simulink model "ccc_core"  (Simulink 7.4)
settings: Solver=ode45  StartTime=0.0  StopTime=10000  RelTol=1e-3
libraries: xbsIndex_r4 x236, cfa_library x64, casper_library_misc x7
(part 2 of 5)

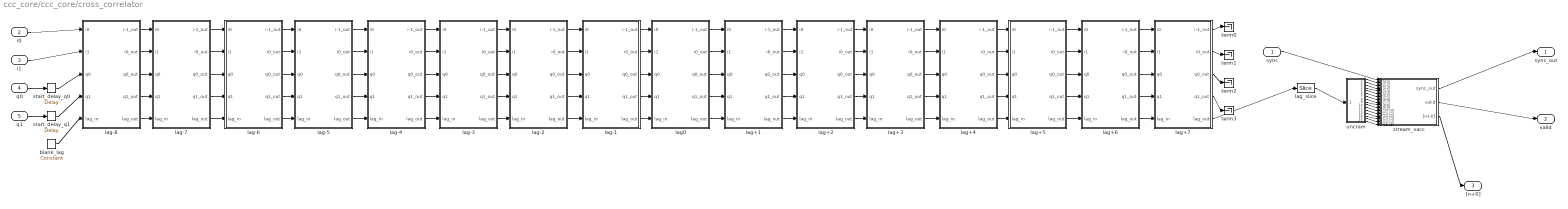
== system ccc_core/ccc_core/cross_correlator ==
  sync : Inport
  i0 : Inport  Port=2
  i1 : Inport  Port=3
  q0 : Inport  Port=4
  q1 : Inport  Port=5
  blank_lag : xbsIndex_r4/Constant  arith_type=Unsigned  const=0  n_bits=1  bin_pt=0  explicit_period=on  period=1  equ=P=C  opselect=C  inp2=PCIN>>17  opr=+  inp1=P  carry=CIN  dbl_ovrd=off  block_type=constant
  lag+1 : Subsystem  AncestorBlock=cfa_library/single_lag  mask(single_lag){n_inputs=1, specify_mult=off, mult_spec=Behavioral, specify_add=off, add_spec=Fabric, mult_delay=3, add_delay=2, overall_delay=2, use_2bit=on, complex_in=on, shift_q=off, shift_i=on}
      mask prompts: n_inputs "Number of Simultaneous Inputs: (2^?)"; specify_mult "Specify multiplier use (behavioural HDL if not specified)"; mult_spec "Multiplier specification:"; specify_add "Specify adder use (behavioural HDL if not specified)"; add_spec "Adder specification:"; mult_delay "Mult Latency:"; add_delay "Add Latency:"; overall_delay "Overall Latency:"; use_2bit "Use special 2-bit binary encoding"; complex_in "Complex inputs"; shift_q "Shift 'q' output"; shift_i "Shift 'i' output"
      mask help: This performs the computations for a single lag. Please use the 'cross_correlator' block to generate a full X-engine.
      mask init:
      | single_lag_init(gcb,...
      |     'n_inputs', n_inputs,...
      |     'specify_mult', specify_mult,...
      |     'mult_spec', mult_spec,...
      |     'specify_add', specify_add,...
      |     'add_spec', add_spec,...
      |     'mult_delay', mult_delay,...
      |     'add_delay', add_delay,...
      |     'overall_delay', overall_delay,...
      |     'use_2bit', use_2bit,...
      |     'complex_in', complex_in,...
      |     'shift_q', shift_q,...
      |     'shift_i', shift_i);
      settings: AttributesFormatString=|
      | Use 2-bit: on, Type: complex,
      |  Demux: 2, Add: Fabric,
      |  Mult: Behavioral
      mask StyleString: edit,checkbox,popup(Behavioral|Core|Embedded),checkbox,popup(Fabric|DSP48),edit,edit,edit,checkbox,checkbox,checkbox,checkbox
      mask CallbackString:
      | |specify_mult = get_param(gcb,'specify_mult');
      | enables = get_param(gcb, 'MaskEnables');
      | if( strcmp(specify_mult,'off')),
      |     enables{3} = 'off';
      | else,
      |     enables{3} = 'on';
      | end
      | set_param(gcb, 'MaskEnables', enables);
      | ||specify_add = get_param(gcb,'specify_add');
      | enables = get_param(gcb, 'MaskEnables');
      | if( strcmp(specify_add,'off')),
      |     enables{5} = 'off';
      | else,
      |     enables{5} = 'on';
      | end
      | set_param(gcb, 'MaskEnables', enables);
      | |||||use_2bit = get_param(gcb,'use_2bit');
      | enables = get_param(gcb, 'MaskEnables');
      | if( strcmp(use_2bit,'off')),
      |     enables{10} = 'off';
      | else,
      |     enables{10} = 'on';
      | end
      | set_param(gcb, 'MaskEnables', enables);|||
      mask TabNameString: Basic,Implementation,Implementation,Implementation,Implementation,Implementation,Implementation,Implementation,Basic,Basic,Basic,Basic
  lag+2 : Subsystem  AncestorBlock=cfa_library/single_lag  mask(single_lag){n_inputs=1, specify_mult=off, mult_spec=Behavioral, specify_add=off, add_spec=Fabric, mult_delay=3, add_delay=2, overall_delay=2, use_2bit=on, complex_in=on, shift_q=off, shift_i=on}
      mask prompts: n_inputs "Number of Simultaneous Inputs: (2^?)"; specify_mult "Specify multiplier use (behavioural HDL if not specified)"; mult_spec "Multiplier specification:"; specify_add "Specify adder use (behavioural HDL if not specified)"; add_spec "Adder specification:"; mult_delay "Mult Latency:"; add_delay "Add Latency:"; overall_delay "Overall Latency:"; use_2bit "Use special 2-bit binary encoding"; complex_in "Complex inputs"; shift_q "Shift 'q' output"; shift_i "Shift 'i' output"
      mask help: This performs the computations for a single lag. Please use the 'cross_correlator' block to generate a full X-engine.
      mask init: same as ccc_core/ccc_core/cross_correlator/lag+1
      settings: AttributesFormatString=|
      | Use 2-bit: on, Type: complex,
      |  Demux: 2, Add: Fabric,
      |  Mult: Behavioral
      mask StyleString: edit,checkbox,popup(Behavioral|Core|Embedded),checkbox,popup(Fabric|DSP48),edit,edit,edit,checkbox,checkbox,checkbox,checkbox
      mask CallbackString:
      | |specify_mult = get_param(gcb,'specify_mult');
      | enables = get_param(gcb, 'MaskEnables');
      | if( strcmp(specify_mult,'off')),
      |     enables{3} = 'off';
      | else,
      |     enables{3} = 'on';
      | end
      | set_param(gcb, 'MaskEnables', enables);
      | ||specify_add = get_param(gcb,'specify_add');
      | enables = get_param(gcb, 'MaskEnables');
      | if( strcmp(specify_add,'off')),
      |     enables{5} = 'off';
      | else,
      |     enables{5} = 'on';
      | end
      | set_param(gcb, 'MaskEnables', enables);
      | |||||use_2bit = get_param(gcb,'use_2bit');
      | enables = get_param(gcb, 'MaskEnables');
      | if( strcmp(use_2bit,'off')),
      |     enables{10} = 'off';
      | else,
      |     enables{10} = 'on';
      | end
      | set_param(gcb, 'MaskEnables', enables);|||
      mask TabNameString: Basic,Implementation,Implementation,Implementation,Implementation,Implementation,Implementation,Implementation,Basic,Basic,Basic,Basic
  lag+3 : Subsystem  AncestorBlock=cfa_library/single_lag  mask(single_lag){n_inputs=1, specify_mult=off, mult_spec=Behavioral, specify_add=off, add_spec=Fabric, mult_delay=3, add_delay=2, overall_delay=2, use_2bit=on, complex_in=on, shift_q=off, shift_i=on}
      mask prompts: n_inputs "Number of Simultaneous Inputs: (2^?)"; specify_mult "Specify multiplier use (behavioural HDL if not specified)"; mult_spec "Multiplier specification:"; specify_add "Specify adder use (behavioural HDL if not specified)"; add_spec "Adder specification:"; mult_delay "Mult Latency:"; add_delay "Add Latency:"; overall_delay "Overall Latency:"; use_2bit "Use special 2-bit binary encoding"; complex_in "Complex inputs"; shift_q "Shift 'q' output"; shift_i "Shift 'i' output"
      mask help: This performs the computations for a single lag. Please use the 'cross_correlator' block to generate a full X-engine.
      mask init: same as ccc_core/ccc_core/cross_correlator/lag+1
      settings: AttributesFormatString=|
      | Use 2-bit: on, Type: complex,
      |  Demux: 2, Add: Fabric,
      |  Mult: Behavioral
      mask StyleString: edit,checkbox,popup(Behavioral|Core|Embedded),checkbox,popup(Fabric|DSP48),edit,edit,edit,checkbox,checkbox,checkbox,checkbox
      mask CallbackString:
      | |specify_mult = get_param(gcb,'specify_mult');
      | enables = get_param(gcb, 'MaskEnables');
      | if( strcmp(specify_mult,'off')),
      |     enables{3} = 'off';
      | else,
      |     enables{3} = 'on';
      | end
      | set_param(gcb, 'MaskEnables', enables);
      | ||specify_add = get_param(gcb,'specify_add');
      | enables = get_param(gcb, 'MaskEnables');
      | if( strcmp(specify_add,'off')),
      |     enables{5} = 'off';
      | else,
      |     enables{5} = 'on';
      | end
      | set_param(gcb, 'MaskEnables', enables);
      | |||||use_2bit = get_param(gcb,'use_2bit');
      | enables = get_param(gcb, 'MaskEnables');
      | if( strcmp(use_2bit,'off')),
      |     enables{10} = 'off';
      | else,
      |     enables{10} = 'on';
      | end
      | set_param(gcb, 'MaskEnables', enables);|||
      mask TabNameString: Basic,Implementation,Implementation,Implementation,Implementation,Implementation,Implementation,Implementation,Basic,Basic,Basic,Basic
  lag+4 : Subsystem  AncestorBlock=cfa_library/single_lag  mask(single_lag){n_inputs=1, specify_mult=off, mult_spec=Behavioral, specify_add=off, add_spec=Fabric, mult_delay=3, add_delay=2, overall_delay=2, use_2bit=on, complex_in=on, shift_q=off, shift_i=on}
      mask prompts: n_inputs "Number of Simultaneous Inputs: (2^?)"; specify_mult "Specify multiplier use (behavioural HDL if not specified)"; mult_spec "Multiplier specification:"; specify_add "Specify adder use (behavioural HDL if not specified)"; add_spec "Adder specification:"; mult_delay "Mult Latency:"; add_delay "Add Latency:"; overall_delay "Overall Latency:"; use_2bit "Use special 2-bit binary encoding"; complex_in "Complex inputs"; shift_q "Shift 'q' output"; shift_i "Shift 'i' output"
      mask help: This performs the computations for a single lag. Please use the 'cross_correlator' block to generate a full X-engine.
      mask init: same as ccc_core/ccc_core/cross_correlator/lag+1
      settings: AttributesFormatString=|
      | Use 2-bit: on, Type: complex,
      |  Demux: 2, Add: Fabric,
      |  Mult: Behavioral
      mask StyleString: edit,checkbox,popup(Behavioral|Core|Embedded),checkbox,popup(Fabric|DSP48),edit,edit,edit,checkbox,checkbox,checkbox,checkbox
      mask CallbackString:
      | |specify_mult = get_param(gcb,'specify_mult');
      | enables = get_param(gcb, 'MaskEnables');
      | if( strcmp(specify_mult,'off')),
      |     enables{3} = 'off';
      | else,
      |     enables{3} = 'on';
      | end
      | set_param(gcb, 'MaskEnables', enables);
      | ||specify_add = get_param(gcb,'specify_add');
      | enables = get_param(gcb, 'MaskEnables');
      | if( strcmp(specify_add,'off')),
      |     enables{5} = 'off';
      | else,
      |     enables{5} = 'on';
      | end
      | set_param(gcb, 'MaskEnables', enables);
      | |||||use_2bit = get_param(gcb,'use_2bit');
      | enables = get_param(gcb, 'MaskEnables');
      | if( strcmp(use_2bit,'off')),
      |     enables{10} = 'off';
      | else,
      |     enables{10} = 'on';
      | end
      | set_param(gcb, 'MaskEnables', enables);|||
      mask TabNameString: Basic,Implementation,Implementation,Implementation,Implementation,Implementation,Implementation,Implementation,Basic,Basic,Basic,Basic
  lag+5 : Subsystem  AncestorBlock=cfa_library/single_lag  mask(single_lag){n_inputs=1, specify_mult=off, mult_spec=Behavioral, specify_add=off, add_spec=Fabric, mult_delay=3, add_delay=2, overall_delay=2, use_2bit=on, complex_in=on, shift_q=off, shift_i=on}
      mask prompts: n_inputs "Number of Simultaneous Inputs: (2^?)"; specify_mult "Specify multiplier use (behavioural HDL if not specified)"; mult_spec "Multiplier specification:"; specify_add "Specify adder use (behavioural HDL if not specified)"; add_spec "Adder specification:"; mult_delay "Mult Latency:"; add_delay "Add Latency:"; overall_delay "Overall Latency:"; use_2bit "Use special 2-bit binary encoding"; complex_in "Complex inputs"; shift_q "Shift 'q' output"; shift_i "Shift 'i' output"
      mask help: This performs the computations for a single lag. Please use the 'cross_correlator' block to generate a full X-engine.
      mask init: same as ccc_core/ccc_core/cross_correlator/lag+1
      settings: AttributesFormatString=|
      | Use 2-bit: on, Type: complex,
      |  Demux: 2, Add: Fabric,
      |  Mult: Behavioral
      mask StyleString: edit,checkbox,popup(Behavioral|Core|Embedded),checkbox,popup(Fabric|DSP48),edit,edit,edit,checkbox,checkbox,checkbox,checkbox
      mask CallbackString:
      | |specify_mult = get_param(gcb,'specify_mult');
      | enables = get_param(gcb, 'MaskEnables');
      | if( strcmp(specify_mult,'off')),
      |     enables{3} = 'off';
      | else,
      |     enables{3} = 'on';
      | end
      | set_param(gcb, 'MaskEnables', enables);
      | ||specify_add = get_param(gcb,'specify_add');
      | enables = get_param(gcb, 'MaskEnables');
      | if( strcmp(specify_add,'off')),
      |     enables{5} = 'off';
      | else,
      |     enables{5} = 'on';
      | end
      | set_param(gcb, 'MaskEnables', enables);
      | |||||use_2bit = get_param(gcb,'use_2bit');
      | enables = get_param(gcb, 'MaskEnables');
      | if( strcmp(use_2bit,'off')),
      |     enables{10} = 'off';
      | else,
      |     enables{10} = 'on';
      | end
      | set_param(gcb, 'MaskEnables', enables);|||
      mask TabNameString: Basic,Implementation,Implementation,Implementation,Implementation,Implementation,Implementation,Implementation,Basic,Basic,Basic,Basic
  lag+6 : Subsystem  AncestorBlock=cfa_library/single_lag  mask(single_lag){n_inputs=1, specify_mult=off, mult_spec=Behavioral, specify_add=off, add_spec=Fabric, mult_delay=3, add_delay=2, overall_delay=2, use_2bit=on, complex_in=on, shift_q=off, shift_i=on}
      mask prompts: n_inputs "Number of Simultaneous Inputs: (2^?)"; specify_mult "Specify multiplier use (behavioural HDL if not specified)"; mult_spec "Multiplier specification:"; specify_add "Specify adder use (behavioural HDL if not specified)"; add_spec "Adder specification:"; mult_delay "Mult Latency:"; add_delay "Add Latency:"; overall_delay "Overall Latency:"; use_2bit "Use special 2-bit binary encoding"; complex_in "Complex inputs"; shift_q "Shift 'q' output"; shift_i "Shift 'i' output"
      mask help: This performs the computations for a single lag. Please use the 'cross_correlator' block to generate a full X-engine.
      mask init: same as ccc_core/ccc_core/cross_correlator/lag+1
      settings: AttributesFormatString=|
      | Use 2-bit: on, Type: complex,
      |  Demux: 2, Add: Fabric,
      |  Mult: Behavioral
      mask StyleString: edit,checkbox,popup(Behavioral|Core|Embedded),checkbox,popup(Fabric|DSP48),edit,edit,edit,checkbox,checkbox,checkbox,checkbox
      mask CallbackString:
      | |specify_mult = get_param(gcb,'specify_mult');
      | enables = get_param(gcb, 'MaskEnables');
      | if( strcmp(specify_mult,'off')),
      |     enables{3} = 'off';
      | else,
      |     enables{3} = 'on';
      | end
      | set_param(gcb, 'MaskEnables', enables);
      | ||specify_add = get_param(gcb,'specify_add');
      | enables = get_param(gcb, 'MaskEnables');
      | if( strcmp(specify_add,'off')),
      |     enables{5} = 'off';
      | else,
      |     enables{5} = 'on';
      | end
      | set_param(gcb, 'MaskEnables', enables);
      | |||||use_2bit = get_param(gcb,'use_2bit');
      | enables = get_param(gcb, 'MaskEnables');
      | if( strcmp(use_2bit,'off')),
      |     enables{10} = 'off';
      | else,
      |     enables{10} = 'on';
      | end
      | set_param(gcb, 'MaskEnables', enables);|||
      mask TabNameString: Basic,Implementation,Implementation,Implementation,Implementation,Implementation,Implementation,Implementation,Basic,Basic,Basic,Basic
  lag+7 : Subsystem  AncestorBlock=cfa_library/single_lag  mask(single_lag){n_inputs=1, specify_mult=off, mult_spec=Behavioral, specify_add=off, add_spec=Fabric, mult_delay=3, add_delay=2, overall_delay=2, use_2bit=on, complex_in=on, shift_q=off, shift_i=on}
      mask prompts: n_inputs "Number of Simultaneous Inputs: (2^?)"; specify_mult "Specify multiplier use (behavioural HDL if not specified)"; mult_spec "Multiplier specification:"; specify_add "Specify adder use (behavioural HDL if not specified)"; add_spec "Adder specification:"; mult_delay "Mult Latency:"; add_delay "Add Latency:"; overall_delay "Overall Latency:"; use_2bit "Use special 2-bit binary encoding"; complex_in "Complex inputs"; shift_q "Shift 'q' output"; shift_i "Shift 'i' output"
      mask help: This performs the computations for a single lag. Please use the 'cross_correlator' block to generate a full X-engine.
      mask init: same as ccc_core/ccc_core/cross_correlator/lag+1
      settings: AttributesFormatString=|
      | Use 2-bit: on, Type: complex,
      |  Demux: 2, Add: Fabric,
      |  Mult: Behavioral
      mask StyleString: edit,checkbox,popup(Behavioral|Core|Embedded),checkbox,popup(Fabric|DSP48),edit,edit,edit,checkbox,checkbox,checkbox,checkbox
      mask CallbackString:
      | |specify_mult = get_param(gcb,'specify_mult');
      | enables = get_param(gcb, 'MaskEnables');
      | if( strcmp(specify_mult,'off')),
      |     enables{3} = 'off';
      | else,
      |     enables{3} = 'on';
      | end
      | set_param(gcb, 'MaskEnables', enables);
      | ||specify_add = get_param(gcb,'specify_add');
      | enables = get_param(gcb, 'MaskEnables');
      | if( strcmp(specify_add,'off')),
      |     enables{5} = 'off';
      | else,
      |     enables{5} = 'on';
      | end
      | set_param(gcb, 'MaskEnables', enables);
      | |||||use_2bit = get_param(gcb,'use_2bit');
      | enables = get_param(gcb, 'MaskEnables');
      | if( strcmp(use_2bit,'off')),
      |     enables{10} = 'off';
      | else,
      |     enables{10} = 'on';
      | end
      | set_param(gcb, 'MaskEnables', enables);|||
      mask TabNameString: Basic,Implementation,Implementation,Implementation,Implementation,Implementation,Implementation,Implementation,Basic,Basic,Basic,Basic
  lag-1 : Subsystem  AncestorBlock=cfa_library/single_lag  mask(single_lag){n_inputs=1, specify_mult=off, mult_spec=Behavioral, specify_add=off, add_spec=Fabric, mult_delay=3, add_delay=2, overall_delay=2, use_2bit=on, complex_in=on, shift_q=off, shift_i=on}
      mask prompts: n_inputs "Number of Simultaneous Inputs: (2^?)"; specify_mult "Specify multiplier use (behavioural HDL if not specified)"; mult_spec "Multiplier specification:"; specify_add "Specify adder use (behavioural HDL if not specified)"; add_spec "Adder specification:"; mult_delay "Mult Latency:"; add_delay "Add Latency:"; overall_delay "Overall Latency:"; use_2bit "Use special 2-bit binary encoding"; complex_in "Complex inputs"; shift_q "Shift 'q' output"; shift_i "Shift 'i' output"
      mask help: This performs the computations for a single lag. Please use the 'cross_correlator' block to generate a full X-engine.
      mask init: same as ccc_core/ccc_core/cross_correlator/lag+1
      settings: AttributesFormatString=|
      | Use 2-bit: on, Type: complex,
      |  Demux: 2, Add: Fabric,
      |  Mult: Behavioral
      mask StyleString: edit,checkbox,popup(Behavioral|Core|Embedded),checkbox,popup(Fabric|DSP48),edit,edit,edit,checkbox,checkbox,checkbox,checkbox
      mask CallbackString:
      | |specify_mult = get_param(gcb,'specify_mult');
      | enables = get_param(gcb, 'MaskEnables');
      | if( strcmp(specify_mult,'off')),
      |     enables{3} = 'off';
      | else,
      |     enables{3} = 'on';
      | end
      | set_param(gcb, 'MaskEnables', enables);
      | ||specify_add = get_param(gcb,'specify_add');
      | enables = get_param(gcb, 'MaskEnables');
      | if( strcmp(specify_add,'off')),
      |     enables{5} = 'off';
      | else,
      |     enables{5} = 'on';
      | end
      | set_param(gcb, 'MaskEnables', enables);
      | |||||use_2bit = get_param(gcb,'use_2bit');
      | enables = get_param(gcb, 'MaskEnables');
      | if( strcmp(use_2bit,'off')),
      |     enables{10} = 'off';
      | else,
      |     enables{10} = 'on';
      | end
      | set_param(gcb, 'MaskEnables', enables);|||
      mask TabNameString: Basic,Implementation,Implementation,Implementation,Implementation,Implementation,Implementation,Implementation,Basic,Basic,Basic,Basic
  lag-2 : Subsystem  AncestorBlock=cfa_library/single_lag  mask(single_lag){n_inputs=1, specify_mult=off, mult_spec=Behavioral, specify_add=off, add_spec=Fabric, mult_delay=3, add_delay=2, overall_delay=2, use_2bit=on, complex_in=on, shift_q=off, shift_i=on}
      mask prompts: n_inputs "Number of Simultaneous Inputs: (2^?)"; specify_mult "Specify multiplier use (behavioural HDL if not specified)"; mult_spec "Multiplier specification:"; specify_add "Specify adder use (behavioural HDL if not specified)"; add_spec "Adder specification:"; mult_delay "Mult Latency:"; add_delay "Add Latency:"; overall_delay "Overall Latency:"; use_2bit "Use special 2-bit binary encoding"; complex_in "Complex inputs"; shift_q "Shift 'q' output"; shift_i "Shift 'i' output"
      mask help: This performs the computations for a single lag. Please use the 'cross_correlator' block to generate a full X-engine.
      mask init: same as ccc_core/ccc_core/cross_correlator/lag+1
      settings: AttributesFormatString=|
      | Use 2-bit: on, Type: complex,
      |  Demux: 2, Add: Fabric,
      |  Mult: Behavioral
      mask StyleString: edit,checkbox,popup(Behavioral|Core|Embedded),checkbox,popup(Fabric|DSP48),edit,edit,edit,checkbox,checkbox,checkbox,checkbox
      mask CallbackString:
      | |specify_mult = get_param(gcb,'specify_mult');
      | enables = get_param(gcb, 'MaskEnables');
      | if( strcmp(specify_mult,'off')),
      |     enables{3} = 'off';
      | else,
      |     enables{3} = 'on';
      | end
      | set_param(gcb, 'MaskEnables', enables);
      | ||specify_add = get_param(gcb,'specify_add');
      | enables = get_param(gcb, 'MaskEnables');
      | if( strcmp(specify_add,'off')),
      |     enables{5} = 'off';
      | else,
      |     enables{5} = 'on';
      | end
      | set_param(gcb, 'MaskEnables', enables);
      | |||||use_2bit = get_param(gcb,'use_2bit');
      | enables = get_param(gcb, 'MaskEnables');
      | if( strcmp(use_2bit,'off')),
      |     enables{10} = 'off';
      | else,
      |     enables{10} = 'on';
      | end
      | set_param(gcb, 'MaskEnables', enables);|||
      mask TabNameString: Basic,Implementation,Implementation,Implementation,Implementation,Implementation,Implementation,Implementation,Basic,Basic,Basic,Basic
  lag-3 : Subsystem  AncestorBlock=cfa_library/single_lag  mask(single_lag){n_inputs=1, specify_mult=off, mult_spec=Behavioral, specify_add=off, add_spec=Fabric, mult_delay=3, add_delay=2, overall_delay=2, use_2bit=on, complex_in=on, shift_q=off, shift_i=on}
      mask prompts: n_inputs "Number of Simultaneous Inputs: (2^?)"; specify_mult "Specify multiplier use (behavioural HDL if not specified)"; mult_spec "Multiplier specification:"; specify_add "Specify adder use (behavioural HDL if not specified)"; add_spec "Adder specification:"; mult_delay "Mult Latency:"; add_delay "Add Latency:"; overall_delay "Overall Latency:"; use_2bit "Use special 2-bit binary encoding"; complex_in "Complex inputs"; shift_q "Shift 'q' output"; shift_i "Shift 'i' output"
      mask help: This performs the computations for a single lag. Please use the 'cross_correlator' block to generate a full X-engine.
      mask init: same as ccc_core/ccc_core/cross_correlator/lag+1
      settings: AttributesFormatString=|
      | Use 2-bit: on, Type: complex,
      |  Demux: 2, Add: Fabric,
      |  Mult: Behavioral
      mask StyleString: edit,checkbox,popup(Behavioral|Core|Embedded),checkbox,popup(Fabric|DSP48),edit,edit,edit,checkbox,checkbox,checkbox,checkbox
      mask CallbackString:
      | |specify_mult = get_param(gcb,'specify_mult');
      | enables = get_param(gcb, 'MaskEnables');
      | if( strcmp(specify_mult,'off')),
      |     enables{3} = 'off';
      | else,
      |     enables{3} = 'on';
      | end
      | set_param(gcb, 'MaskEnables', enables);
      | ||specify_add = get_param(gcb,'specify_add');
      | enables = get_param(gcb, 'MaskEnables');
      | if( strcmp(specify_add,'off')),
      |     enables{5} = 'off';
      | else,
      |     enables{5} = 'on';
      | end
      | set_param(gcb, 'MaskEnables', enables);
      | |||||use_2bit = get_param(gcb,'use_2bit');
      | enables = get_param(gcb, 'MaskEnables');
      | if( strcmp(use_2bit,'off')),
      |     enables{10} = 'off';
      | else,
      |     enables{10} = 'on';
      | end
      | set_param(gcb, 'MaskEnables', enables);|||
      mask TabNameString: Basic,Implementation,Implementation,Implementation,Implementation,Implementation,Implementation,Implementation,Basic,Basic,Basic,Basic
  lag-4 : Subsystem  AncestorBlock=cfa_library/single_lag  mask(single_lag){n_inputs=1, specify_mult=off, mult_spec=Behavioral, specify_add=off, add_spec=Fabric, mult_delay=3, add_delay=2, overall_delay=2, use_2bit=on, complex_in=on, shift_q=off, shift_i=on}
      mask prompts: n_inputs "Number of Simultaneous Inputs: (2^?)"; specify_mult "Specify multiplier use (behavioural HDL if not specified)"; mult_spec "Multiplier specification:"; specify_add "Specify adder use (behavioural HDL if not specified)"; add_spec "Adder specification:"; mult_delay "Mult Latency:"; add_delay "Add Latency:"; overall_delay "Overall Latency:"; use_2bit "Use special 2-bit binary encoding"; complex_in "Complex inputs"; shift_q "Shift 'q' output"; shift_i "Shift 'i' output"
      mask help: This performs the computations for a single lag. Please use the 'cross_correlator' block to generate a full X-engine.
      mask init: same as ccc_core/ccc_core/cross_correlator/lag+1
      settings: AttributesFormatString=|
      | Use 2-bit: on, Type: complex,
      |  Demux: 2, Add: Fabric,
      |  Mult: Behavioral
      mask StyleString: edit,checkbox,popup(Behavioral|Core|Embedded),checkbox,popup(Fabric|DSP48),edit,edit,edit,checkbox,checkbox,checkbox,checkbox
      mask CallbackString:
      | |specify_mult = get_param(gcb,'specify_mult');
      | enables = get_param(gcb, 'MaskEnables');
      | if( strcmp(specify_mult,'off')),
      |     enables{3} = 'off';
      | else,
      |     enables{3} = 'on';
      | end
      | set_param(gcb, 'MaskEnables', enables);
      | ||specify_add = get_param(gcb,'specify_add');
      | enables = get_param(gcb, 'MaskEnables');
      | if( strcmp(specify_add,'off')),
      |     enables{5} = 'off';
      | else,
      |     enables{5} = 'on';
      | end
      | set_param(gcb, 'MaskEnables', enables);
      | |||||use_2bit = get_param(gcb,'use_2bit');
      | enables = get_param(gcb, 'MaskEnables');
      | if( strcmp(use_2bit,'off')),
      |     enables{10} = 'off';
      | else,
      |     enables{10} = 'on';
      | end
      | set_param(gcb, 'MaskEnables', enables);|||
      mask TabNameString: Basic,Implementation,Implementation,Implementation,Implementation,Implementation,Implementation,Implementation,Basic,Basic,Basic,Basic
  lag-5 : Subsystem  AncestorBlock=cfa_library/single_lag  mask(single_lag){n_inputs=1, specify_mult=off, mult_spec=Behavioral, specify_add=off, add_spec=Fabric, mult_delay=3, add_delay=2, overall_delay=2, use_2bit=on, complex_in=on, shift_q=off, shift_i=on}
      mask prompts: n_inputs "Number of Simultaneous Inputs: (2^?)"; specify_mult "Specify multiplier use (behavioural HDL if not specified)"; mult_spec "Multiplier specification:"; specify_add "Specify adder use (behavioural HDL if not specified)"; add_spec "Adder specification:"; mult_delay "Mult Latency:"; add_delay "Add Latency:"; overall_delay "Overall Latency:"; use_2bit "Use special 2-bit binary encoding"; complex_in "Complex inputs"; shift_q "Shift 'q' output"; shift_i "Shift 'i' output"
      mask help: This performs the computations for a single lag. Please use the 'cross_correlator' block to generate a full X-engine.
      mask init: same as ccc_core/ccc_core/cross_correlator/lag+1
      settings: AttributesFormatString=|
      | Use 2-bit: on, Type: complex,
      |  Demux: 2, Add: Fabric,
      |  Mult: Behavioral
      mask StyleString: edit,checkbox,popup(Behavioral|Core|Embedded),checkbox,popup(Fabric|DSP48),edit,edit,edit,checkbox,checkbox,checkbox,checkbox
      mask CallbackString:
      | |specify_mult = get_param(gcb,'specify_mult');
      | enables = get_param(gcb, 'MaskEnables');
      | if( strcmp(specify_mult,'off')),
      |     enables{3} = 'off';
      | else,
      |     enables{3} = 'on';
      | end
      | set_param(gcb, 'MaskEnables', enables);
      | ||specify_add = get_param(gcb,'specify_add');
      | enables = get_param(gcb, 'MaskEnables');
      | if( strcmp(specify_add,'off')),
      |     enables{5} = 'off';
      | else,
      |     enables{5} = 'on';
      | end
      | set_param(gcb, 'MaskEnables', enables);
      | |||||use_2bit = get_param(gcb,'use_2bit');
      | enables = get_param(gcb, 'MaskEnables');
      | if( strcmp(use_2bit,'off')),
      |     enables{10} = 'off';
      | else,
      |     enables{10} = 'on';
      | end
      | set_param(gcb, 'MaskEnables', enables);|||
      mask TabNameString: Basic,Implementation,Implementation,Implementation,Implementation,Implementation,Implementation,Implementation,Basic,Basic,Basic,Basic
  lag-6 : Subsystem  AncestorBlock=cfa_library/single_lag  mask(single_lag){n_inputs=1, specify_mult=off, mult_spec=Behavioral, specify_add=off, add_spec=Fabric, mult_delay=3, add_delay=2, overall_delay=2, use_2bit=on, complex_in=on, shift_q=off, shift_i=on}
      mask prompts: n_inputs "Number of Simultaneous Inputs: (2^?)"; specify_mult "Specify multiplier use (behavioural HDL if not specified)"; mult_spec "Multiplier specification:"; specify_add "Specify adder use (behavioural HDL if not specified)"; add_spec "Adder specification:"; mult_delay "Mult Latency:"; add_delay "Add Latency:"; overall_delay "Overall Latency:"; use_2bit "Use special 2-bit binary encoding"; complex_in "Complex inputs"; shift_q "Shift 'q' output"; shift_i "Shift 'i' output"
      mask help: This performs the computations for a single lag. Please use the 'cross_correlator' block to generate a full X-engine.
      mask init: same as ccc_core/ccc_core/cross_correlator/lag+1
      settings: AttributesFormatString=|
      | Use 2-bit: on, Type: complex,
      |  Demux: 2, Add: Fabric,
      |  Mult: Behavioral
      mask StyleString: edit,checkbox,popup(Behavioral|Core|Embedded),checkbox,popup(Fabric|DSP48),edit,edit,edit,checkbox,checkbox,checkbox,checkbox
      mask CallbackString:
      | |specify_mult = get_param(gcb,'specify_mult');
      | enables = get_param(gcb, 'MaskEnables');
      | if( strcmp(specify_mult,'off')),
      |     enables{3} = 'off';
      | else,
      |     enables{3} = 'on';
      | end
      | set_param(gcb, 'MaskEnables', enables);
      | ||specify_add = get_param(gcb,'specify_add');
      | enables = get_param(gcb, 'MaskEnables');
      | if( strcmp(specify_add,'off')),
      |     enables{5} = 'off';
      | else,
      |     enables{5} = 'on';
      | end
      | set_param(gcb, 'MaskEnables', enables);
      | |||||use_2bit = get_param(gcb,'use_2bit');
      | enables = get_param(gcb, 'MaskEnables');
      | if( strcmp(use_2bit,'off')),
      |     enables{10} = 'off';
      | else,
      |     enables{10} = 'on';
      | end
      | set_param(gcb, 'MaskEnables', enables);|||
      mask TabNameString: Basic,Implementation,Implementation,Implementation,Implementation,Implementation,Implementation,Implementation,Basic,Basic,Basic,Basic
  lag-7 : Subsystem  AncestorBlock=cfa_library/single_lag  mask(single_lag){n_inputs=1, specify_mult=off, mult_spec=Behavioral, specify_add=off, add_spec=Fabric, mult_delay=3, add_delay=2, overall_delay=2, use_2bit=on, complex_in=on, shift_q=off, shift_i=on}
      mask prompts: n_inputs "Number of Simultaneous Inputs: (2^?)"; specify_mult "Specify multiplier use (behavioural HDL if not specified)"; mult_spec "Multiplier specification:"; specify_add "Specify adder use (behavioural HDL if not specified)"; add_spec "Adder specification:"; mult_delay "Mult Latency:"; add_delay "Add Latency:"; overall_delay "Overall Latency:"; use_2bit "Use special 2-bit binary encoding"; complex_in "Complex inputs"; shift_q "Shift 'q' output"; shift_i "Shift 'i' output"
      mask help: This performs the computations for a single lag. Please use the 'cross_correlator' block to generate a full X-engine.
      mask init: same as ccc_core/ccc_core/cross_correlator/lag+1
      settings: AttributesFormatString=|
      | Use 2-bit: on, Type: complex,
      |  Demux: 2, Add: Fabric,
      |  Mult: Behavioral
      mask StyleString: edit,checkbox,popup(Behavioral|Core|Embedded),checkbox,popup(Fabric|DSP48),edit,edit,edit,checkbox,checkbox,checkbox,checkbox
      mask CallbackString:
      | |specify_mult = get_param(gcb,'specify_mult');
      | enables = get_param(gcb, 'MaskEnables');
      | if( strcmp(specify_mult,'off')),
      |     enables{3} = 'off';
      | else,
      |     enables{3} = 'on';
      | end
      | set_param(gcb, 'MaskEnables', enables);
      | ||specify_add = get_param(gcb,'specify_add');
      | enables = get_param(gcb, 'MaskEnables');
      | if( strcmp(specify_add,'off')),
      |     enables{5} = 'off';
      | else,
      |     enables{5} = 'on';
      | end
      | set_param(gcb, 'MaskEnables', enables);
      | |||||use_2bit = get_param(gcb,'use_2bit');
      | enables = get_param(gcb, 'MaskEnables');
      | if( strcmp(use_2bit,'off')),
      |     enables{10} = 'off';
      | else,
      |     enables{10} = 'on';
      | end
      | set_param(gcb, 'MaskEnables', enables);|||
      mask TabNameString: Basic,Implementation,Implementation,Implementation,Implementation,Implementation,Implementation,Implementation,Basic,Basic,Basic,Basic
  lag-8 : Subsystem  AncestorBlock=cfa_library/single_lag  mask(single_lag){n_inputs=1, specify_mult=off, mult_spec=Behavioral, specify_add=off, add_spec=Fabric, mult_delay=3, add_delay=2, overall_delay=2, use_2bit=on, complex_in=on, shift_q=off, shift_i=on}
      mask prompts: n_inputs "Number of Simultaneous Inputs: (2^?)"; specify_mult "Specify multiplier use (behavioural HDL if not specified)"; mult_spec "Multiplier specification:"; specify_add "Specify adder use (behavioural HDL if not specified)"; add_spec "Adder specification:"; mult_delay "Mult Latency:"; add_delay "Add Latency:"; overall_delay "Overall Latency:"; use_2bit "Use special 2-bit binary encoding"; complex_in "Complex inputs"; shift_q "Shift 'q' output"; shift_i "Shift 'i' output"
      mask help: This performs the computations for a single lag. Please use the 'cross_correlator' block to generate a full X-engine.
      mask init: same as ccc_core/ccc_core/cross_correlator/lag+1
      settings: AttributesFormatString=|
      | Use 2-bit: on, Type: complex,
      |  Demux: 2, Add: Fabric,
      |  Mult: Behavioral
      mask StyleString: edit,checkbox,popup(Behavioral|Core|Embedded),checkbox,popup(Fabric|DSP48),edit,edit,edit,checkbox,checkbox,checkbox,checkbox
      mask CallbackString:
      | |specify_mult = get_param(gcb,'specify_mult');
      | enables = get_param(gcb, 'MaskEnables');
      | if( strcmp(specify_mult,'off')),
      |     enables{3} = 'off';
      | else,
      |     enables{3} = 'on';
      | end
      | set_param(gcb, 'MaskEnables', enables);
      | ||specify_add = get_param(gcb,'specify_add');
      | enables = get_param(gcb, 'MaskEnables');
      | if( strcmp(specify_add,'off')),
      |     enables{5} = 'off';
      | else,
      |     enables{5} = 'on';
      | end
      | set_param(gcb, 'MaskEnables', enables);
      | |||||use_2bit = get_param(gcb,'use_2bit');
      | enables = get_param(gcb, 'MaskEnables');
      | if( strcmp(use_2bit,'off')),
      |     enables{10} = 'off';
      | else,
      |     enables{10} = 'on';
      | end
      | set_param(gcb, 'MaskEnables', enables);|||
      mask TabNameString: Basic,Implementation,Implementation,Implementation,Implementation,Implementation,Implementation,Implementation,Basic,Basic,Basic,Basic
  lag0 : Subsystem  AncestorBlock=cfa_library/single_lag  mask(single_lag){n_inputs=1, specify_mult=off, mult_spec=Behavioral, specify_add=off, add_spec=Fabric, mult_delay=3, add_delay=2, overall_delay=2, use_2bit=on, complex_in=on, shift_q=off, shift_i=on}
      mask prompts: n_inputs "Number of Simultaneous Inputs: (2^?)"; specify_mult "Specify multiplier use (behavioural HDL if not specified)"; mult_spec "Multiplier specification:"; specify_add "Specify adder use (behavioural HDL if not specified)"; add_spec "Adder specification:"; mult_delay "Mult Latency:"; add_delay "Add Latency:"; overall_delay "Overall Latency:"; use_2bit "Use special 2-bit binary encoding"; complex_in "Complex inputs"; shift_q "Shift 'q' output"; shift_i "Shift 'i' output"
      mask help: This performs the computations for a single lag. Please use the 'cross_correlator' block to generate a full X-engine.
      mask init: same as ccc_core/ccc_core/cross_correlator/lag+1
      settings: AttributesFormatString=|
      | Use 2-bit: on, Type: complex,
      |  Demux: 2, Add: Fabric,
      |  Mult: Behavioral
      mask StyleString: edit,checkbox,popup(Behavioral|Core|Embedded),checkbox,popup(Fabric|DSP48),edit,edit,edit,checkbox,checkbox,checkbox,checkbox
      mask CallbackString:
      | |specify_mult = get_param(gcb,'specify_mult');
      | enables = get_param(gcb, 'MaskEnables');
      | if( strcmp(specify_mult,'off')),
      |     enables{3} = 'off';
      | else,
      |     enables{3} = 'on';
      | end
      | set_param(gcb, 'MaskEnables', enables);
      | ||specify_add = get_param(gcb,'specify_add');
      | enables = get_param(gcb, 'MaskEnables');
      | if( strcmp(specify_add,'off')),
      |     enables{5} = 'off';
      | else,
      |     enables{5} = 'on';
      | end
      | set_param(gcb, 'MaskEnables', enables);
      | |||||use_2bit = get_param(gcb,'use_2bit');
      | enables = get_param(gcb, 'MaskEnables');
      | if( strcmp(use_2bit,'off')),
      |     enables{10} = 'off';
      | else,
      |     enables{10} = 'on';
      | end
      | set_param(gcb, 'MaskEnables', enables);|||
      mask TabNameString: Basic,Implementation,Implementation,Implementation,Implementation,Implementation,Implementation,Implementation,Basic,Basic,Basic,Basic
  lag_slice : xbsIndex_r4/Slice  nbits=224  boolean_output=off  mode=Lower Bit Location + Width  bit1=0  base1=MSB of Input  bit0=0  base0=LSB of Input  dbl_ovrd=off  block_type=slice
      settings: infoedit="Extracts a given range of bits from each input sample and presents it at the output.  The output type is ordinarily unsigned with binary point at zero, but can be Boolean when the slice is one bit wide.<P><P>Hardware notes: In hardware this block costs nothing."  block_version=10.1.3
  start_delay_q0 : xbsIndex_r4/Delay  en=off  latency=4  dbl_ovrd=off  reg_retiming=off  block_type=delay
  start_delay_q1 : xbsIndex_r4/Delay  en=off  latency=4  dbl_ovrd=off  reg_retiming=off  block_type=delay
  stream_vacc : Subsystem  AncestorBlock=cfa_library/stream_vacc  mask(stream_vacc){vector_len=4, input_bit_width=7, input_bin_pt=0, complex_in=on, samples_out=0, output_bit_width=11, output_bin_pt=0, quantization=Truncate, overflow=Wrap, specify_add=off, add_spec=Fabric, add_delay=1}
      mask prompts: vector_len "Vector Length: (2^?)"; input_bit_width "Input Bit Width:"; input_bin_pt "Input Binary Point:"; complex_in "Complex inputs"; samples_out "Number of Simultaneous Outputs: (2^?)"; output_bit_width "Output Bit Width:"; output_bin_pt "Output Binary Point:"; quantization "Quantization Behavior:"; overflow "Overflow Behavior:"; specify_add "Specify adder use (behavioural HDL if not specified)"; add_spec "Adder specification:"; add_delay "Add Latency:"
      mask help: This block implements the second stage adder for the cross_correlator block.
      mask init:
      | stream_vacc_init(gcb,...
      |     'vector_len', vector_len,...
      |     'input_bit_width', input_bit_width,...
      |     'input_bin_pt', input_bin_pt,...
      |     'complex_in', complex_in,...
      |     'samples_out', samples_out,...
      |     'output_bit_width', output_bit_width,...
      |     'output_bin_pt', output_bin_pt,...
      |     'quantization', quantization,...
      |     'overflow', overflow,...
      |     'specify_add', specify_add,...
      |     'add_spec', add_spec,...
      |     'add_delay', add_delay);
      settings: AttributesFormatString=|
      | 16=>1 complex samples
      | Accumulate
      mask StyleString: edit,edit,edit,checkbox,edit,edit,edit,popup(Truncate|Round  (unbiased: +/- Inf)),popup(Wrap|Saturate|Flag as error),checkbox,popup(Fabric|DSP48),edit
      mask CallbackString:
      | ||||vector_len = str2num(get_param(gcb, 'vector_len'));
      | samples_out = str2num(get_param(gcb, 'samples_out'));
      | 
      | if vector_len<samples_out,
      |     error('Number of parallel streams must be greater than or equal to the vector length!');
      | end|||||specify_add = get_param(gcb,'specify_add');
      | enables = get_param(gcb, 'MaskEnables');
      | if( strcmp(specify_add,'off')),
      |     enables{11} = 'off';
      | else
      |     enables{11} = 'on';
      | end
      | set_param(gcb, 'MaskEnables', enables);||
      mask TabNameString: Basic,Input,Input,Input,Basic,Output,Output,Output,Output,Implementation,Implementation,Implementation
  term{0..3} (4 alike) : Terminator
  uncram : Subsystem  AncestorBlock=gavrt_library/uncram  mask(uncram){num_slice=16, slice_width=14, bin_pt=0, arith_type=0}
      mask prompts: num_slice "Number of slices"; slice_width "Slice Width"; bin_pt "Output Binary Point"; arith_type "Output Arithmetic Type (0=Unsigned, 1=Signed)"
      mask help: Takes a concatenated input and slices it up into even pieces and reinterprets them as signed fixed point numbers with a given binary point.
      mask init:
      | uncram_init(gcb, ...
      |     'num_slice', num_slice, ...
      |     'slice_width', slice_width, ...
      |     'bin_pt', bin_pt, ...
      |     'arith_type', arith_type);
      settings: AttributesFormatString=UFix_14_0
  sync_out : Outport
  valid : Outport  Port=2
  "[n+0]" : Outport  Port=3
  wires:
  q0/1 -> start_delay_q0/1
  q1/1 -> start_delay_q1/1
  blank_lag/1 -> lag-8/5(lag_in)
  i0/1 -> lag-8/1(i0)
  start_delay_q0/1 -> lag-8/3(q0)
  i1/1 -> lag-8/2(i1)
  start_delay_q1/1 -> lag-8/4(q1)
  lag-8/1(i-1_out) -> lag-7/1(i0)
  lag-8/2(i0_out) -> lag-7/2(i1)
  lag-8/3(q0_out) -> lag-7/3(q0)
  lag-8/4(q1_out) -> lag-7/4(q1)
  lag-8/5(lag_out) -> lag-7/5(lag_in)
  lag-7/1(i-1_out) -> lag-6/1(i0)
  lag-7/2(i0_out) -> lag-6/2(i1)
  lag-7/3(q0_out) -> lag-6/3(q0)
  lag-7/4(q1_out) -> lag-6/4(q1)
  lag-7/5(lag_out) -> lag-6/5(lag_in)
  lag-6/1(i-1_out) -> lag-5/1(i0)
  lag-6/2(i0_out) -> lag-5/2(i1)
  lag-6/3(q0_out) -> lag-5/3(q0)
  lag-6/4(q1_out) -> lag-5/4(q1)
  lag-6/5(lag_out) -> lag-5/5(lag_in)
  lag-5/1(i-1_out) -> lag-4/1(i0)
  lag-5/2(i0_out) -> lag-4/2(i1)
  lag-5/3(q0_out) -> lag-4/3(q0)
  lag-5/4(q1_out) -> lag-4/4(q1)
  lag-5/5(lag_out) -> lag-4/5(lag_in)
  lag-4/1(i-1_out) -> lag-3/1(i0)
  lag-4/2(i0_out) -> lag-3/2(i1)
  lag-4/3(q0_out) -> lag-3/3(q0)
  lag-4/4(q1_out) -> lag-3/4(q1)
  lag-4/5(lag_out) -> lag-3/5(lag_in)
  lag-3/1(i-1_out) -> lag-2/1(i0)
  lag-3/2(i0_out) -> lag-2/2(i1)
  lag-3/3(q0_out) -> lag-2/3(q0)
  lag-3/4(q1_out) -> lag-2/4(q1)
  lag-3/5(lag_out) -> lag-2/5(lag_in)
  lag-2/1(i-1_out) -> lag-1/1(i0)
  lag-2/2(i0_out) -> lag-1/2(i1)
  lag-2/3(q0_out) -> lag-1/3(q0)
  lag-2/4(q1_out) -> lag-1/4(q1)
  lag-2/5(lag_out) -> lag-1/5(lag_in)
  lag-1/1(i-1_out) -> lag0/1(i0)
  lag-1/2(i0_out) -> lag0/2(i1)
  lag-1/3(q0_out) -> lag0/3(q0)
  lag-1/4(q1_out) -> lag0/4(q1)
  lag-1/5(lag_out) -> lag0/5(lag_in)
  lag0/1(i-1_out) -> lag+1/1(i0)
  lag0/2(i0_out) -> lag+1/2(i1)
  lag0/3(q0_out) -> lag+1/3(q0)
  lag0/4(q1_out) -> lag+1/4(q1)
  lag0/5(lag_out) -> lag+1/5(lag_in)
  lag+1/1(i-1_out) -> lag+2/1(i0)
  lag+1/2(i0_out) -> lag+2/2(i1)
  lag+1/3(q0_out) -> lag+2/3(q0)
  lag+1/4(q1_out) -> lag+2/4(q1)
  lag+1/5(lag_out) -> lag+2/5(lag_in)
  lag+2/1(i-1_out) -> lag+3/1(i0)
  lag+2/2(i0_out) -> lag+3/2(i1)
  lag+2/3(q0_out) -> lag+3/3(q0)
  lag+2/4(q1_out) -> lag+3/4(q1)
  lag+2/5(lag_out) -> lag+3/5(lag_in)
  lag+3/1(i-1_out) -> lag+4/1(i0)
  lag+3/2(i0_out) -> lag+4/2(i1)
  lag+3/3(q0_out) -> lag+4/3(q0)
  lag+3/4(q1_out) -> lag+4/4(q1)
  lag+3/5(lag_out) -> lag+4/5(lag_in)
  lag+4/1(i-1_out) -> lag+5/1(i0)
  lag+4/2(i0_out) -> lag+5/2(i1)
  lag+4/3(q0_out) -> lag+5/3(q0)
  lag+4/4(q1_out) -> lag+5/4(q1)
  lag+4/5(lag_out) -> lag+5/5(lag_in)
  lag+5/1(i-1_out) -> lag+6/1(i0)
  lag+5/2(i0_out) -> lag+6/2(i1)
  lag+5/3(q0_out) -> lag+6/3(q0)
  lag+5/4(q1_out) -> lag+6/4(q1)
  lag+5/5(lag_out) -> lag+6/5(lag_in)
  lag+6/1(i-1_out) -> lag+7/1(i0)
  lag+6/2(i0_out) -> lag+7/2(i1)
  lag+6/3(q0_out) -> lag+7/3(q0)
  lag+6/4(q1_out) -> lag+7/4(q1)
  lag+6/5(lag_out) -> lag+7/5(lag_in)
  lag+7/1(i-1_out) -> term0/1
  lag+7/2(i0_out) -> term1/1
  lag+7/3(q0_out) -> term2/1
  lag+7/4(q1_out) -> term3/1
  lag+7/5(lag_out) -> lag_slice/1
  lag_slice/1 -> uncram/1(In)
  sync/1 -> stream_vacc/1(sync)
  uncram/1(Out1) -> stream_vacc/2("[0-0]")
  uncram/2(Out2) -> stream_vacc/3("[1-1]")
  uncram/3(Out3) -> stream_vacc/4("[2-2]")
  uncram/4(Out4) -> stream_vacc/5("[3-3]")
  uncram/5(Out5) -> stream_vacc/6("[4-4]")
  uncram/6(Out6) -> stream_vacc/7("[5-5]")
  uncram/7(Out7) -> stream_vacc/8("[6-6]")
  uncram/8(Out8) -> stream_vacc/9("[7-7]")
  uncram/9(Out9) -> stream_vacc/10("[8-8]")
  uncram/10(Out10) -> stream_vacc/11("[9-9]")
  uncram/11(Out11) -> stream_vacc/12("[10-10]")
  uncram/12(Out12) -> stream_vacc/13("[11-11]")
  uncram/13(Out13) -> stream_vacc/14("[12-12]")
  uncram/14(Out14) -> stream_vacc/15("[13-13]")
  uncram/15(Out15) -> stream_vacc/16("[14-14]")
  uncram/16(Out16) -> stream_vacc/17("[15-15]")
  stream_vacc/1(sync_out) -> sync_out/1
  stream_vacc/2(valid) -> valid/1
  stream_vacc/3("[n+0]") -> "[n+0]"/1

== system ccc_core/ccc_core/ctrl ==
  integ_time : Inport
  Delay8 : xbsIndex_r4/Delay  en=off  latency=1  dbl_ovrd=off  reg_retiming=off  block_type=delay
      settings: block_version=11.4
  Logical : xbsIndex_r4/Logical  logical_function=OR  inputs=2  en=off  latency=0  precision=Full  arith_type=Unsigned  n_bits=16  bin_pt=0  align_bp=on  dbl_ovrd=off  block_type=logical
      settings: block_version=11.4
  Relational : xbsIndex_r4/Relational  mode=a<=b  en=off  latency=1  dbl_ovrd=off  block_type=relational
  frame_cntr : xbsIndex_r4/Counter  cnt_type=Free Running  cnt_to=Inf  operation=Up  start_count=0  cnt_by_val=1  arith_type=Unsigned  n_bits=32  bin_pt=0  load_pin=off  rst=on  en=on  explicit_period=on  period=1  dbl_ovrd=off  use_behavioral_HDL=off  implementation=Fabric  use_rpm=off  block_type=counter
      settings: block_version=11.4
  integ_cntr : xbsIndex_r4/Counter  cnt_type=Free Running  cnt_to=Inf  operation=Up  start_count=0  cnt_by_val=1  arith_type=Unsigned  n_bits=32  bin_pt=0  load_pin=off  rst=off  en=on  explicit_period=on  period=1  dbl_ovrd=off  use_behavioral_HDL=off  implementation=Fabric  use_rpm=off  block_type=counter
      settings: block_version=11.4
  lag_cntr : xbsIndex_r4/Counter  cnt_type=Free Running  cnt_to=Inf  operation=Up  start_count=0  cnt_by_val=1  arith_type=Unsigned  n_bits=total_lags  bin_pt=0  load_pin=off  rst=on  en=off  explicit_period=on  period=1  dbl_ovrd=off  use_behavioral_HDL=off  implementation=Fabric  use_rpm=off  block_type=counter
      settings: block_version=11.4
  posedge1 : casper_library_misc/posedge  Tag=Rising Edge Detector  SystemSampleTime=-1
  integs : Outport
  tag scope: frames=global, lags=global, new_acc=global
  wires:
  frame_cntr/1 -> Relational/2, [frames]
  Logical/1 -> frame_cntr/1
  Relational/1 -> posedge1/1
  posedge1/1 -> Logical/1, integ_cntr/1, [new_acc]
  integ_time/1 -> Relational/1
  integ_cntr/1 -> integs/1
  lag_cntr/1 -> Delay8/1
  [sync_out] -> Logical/2, lag_cntr/1
  [valid_out] -> frame_cntr/2
  Delay8/1 -> [lags]

== system ccc_core/ccc_core/imag_bram_vacc ==
  new_acc : Inport  OutDataType=sfix(16)  OutScaling=2^0
  din : Inport  Port=2  OutDataType=sfix(16)  OutScaling=2^0
  Adder : xbsIndex_r4/AddSub  mode=Addition  use_carryin=off  use_carryout=off  en=off  latency=add_latency  precision=User Defined  arith_type="Signed  (2's comp)"  n_bits=n_bits  bin_pt=bin_pt  quantization=Truncate  overflow=Wrap  dbl_ovrd=off  use_behavioral_HDL=off  hw_selection=Fabric  pipelined=on  use_rpm=on  block_type=addsub
      settings: xl_area=[0, 0, 0, 0, 0, 0, 0]  block_version=10.1.3
  Constant : xbsIndex_r4/Constant  arith_type=Signed (2's comp)  const=0  n_bits=n_bits  bin_pt=bin_pt  explicit_period=on  period=1  equ=P=C  opselect=C  inp2=PCIN>>17  opr=+  inp1=P  carry=CIN  dbl_ovrd=off  block_type=constant
  Mux : xbsIndex_r4/Mux  inputs=2  en=off  latency=0  precision=Full  arith_type="Signed  (2's comp)"  n_bits=8  bin_pt=2  quantization=Truncate  overflow=Wrap  dbl_ovrd=off  block_type=mux
      settings: xl_area=[0, 0, 0, 0, 0, 0, 0]
  delay_bram : Subsystem  mask(delay_bram){DelayLen=vec_len - add_latency, bram_latency=add_latency}
      mask prompts: DelayLen "Delay By:"; bram_latency "BRAM Latency"
      mask help: A delay block that uses BRAM for its storage.
      mask init:
      | if (DelayLen <= bram_latency)
      | 	error('delay value must be greater than BRAM Latency');
      | end
      | BitWidth = max(ceil(log2(DelayLen)), 2);
      mask Help: eval('xlWeb(''http://casper.berkeley.edu/wiki/Delay_bram'')')
  pulse_ext : Subsystem  mask(pulse_ext){pulse_len=vec_len}
      mask prompts: pulse_len "Length of Pulse"
      mask help:
      | Extends a boolean signal to be high for the specified number of clocks after
      | the last high input.
      mask init:
      | bits = ceil(log2(pulse_len+1));
      mask Help: eval('xlWeb(''http://casper.berkeley.edu/wiki/Pulse_ext'')')
  dout : Outport  OutDataType=sfix(16)  OutScaling=2^0
  valid : Outport  Port=2  OutDataType=sfix(16)  OutScaling=2^0
  wires:
  Constant/1 -> Mux/3
  Mux/1 -> Adder/2
  pulse_ext/1(out) -> valid/1, Mux/1
  din/1 -> Adder/1
  new_acc/1 -> pulse_ext/1(in)
  delay_bram/1(Out1) -> Mux/2, dout/1
  Adder/1 -> delay_bram/1(In1)
